simulink model "WWB_G1_acs"  (R2016a)
settings: Solver=VariableStepAuto  SolverMode=SingleTasking  StartTime=0.0  StopTime=10  RelTol=1e-3
values from neighbouring files (symbols this model uses):
  dendz = sym2poly(D)    [WWB_G1_STEP.m]    (also in WWB_G1_V.m; WWB_G1_ac.m; step_YWB_G1.m)
  numdz = sym2poly(N)    [WWB_G1_STEP.m]    (also in WWB_G1_V.m; WWB_G1_ac.m; step_YWB_G1.m)
libraries: simulink x1
settings Model: Creator=Fish_Schrodinger  LastModifiedBy=Fish_Schrodinger
settings DataIOCC: LimitDataPoints=on  SaveOutput=off  SaveTime=off
settings OptimizationCC: BlockReduction=off  BooleanDataType=off
settings DebuggingCC: SaveWithParameterizedLinksMsg=none  UnderspecifiedInitializationDetection=Classic  MergeDetectMultiDrivingBlocksExec=none  SignalResolutionControl=TryResolveAllWithWarning  AllowSymbolicDim=off
settings HardwareCC: TargetUnknown=on

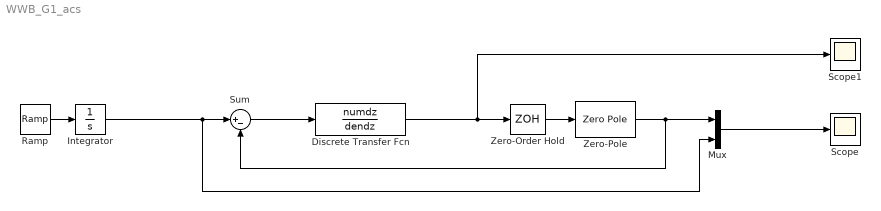
== system WWB_G1_acs ==
  Discrete Transfer Fcn : DiscreteTransferFcn  Numerator=numdz  Denominator=dendz  SampleTime=0.5
  Integrator : Integrator
  Mux : Mux  Inputs=2
  Ramp : simulink/Sources/Ramp  slope=1  start=0  X0=0
  Scope : Scope
  Scope1 : Scope
  Sum : Sum  Inputs=|+-
  Zero-Order Hold : ZeroOrderHold  SampleTime=0.5
  Zero-Pole : ZeroPole  Zeros=[]  Poles=[0 -2]  Gain=[2]
  wires:
  Sum/1 -> Discrete Transfer Fcn/1
  Discrete Transfer Fcn/1 -> Scope1/1, Zero-Order Hold/1
  Zero-Order Hold/1 -> Zero-Pole/1
  Zero-Pole/1 -> Mux/1, Sum/2
  Integrator/1 -> Mux/2, Sum/1
  Mux/1 -> Scope/1
  Ramp/1 -> Integrator/1
